simulink model "MiMo_Sim"  (R2014a)
settings: Solver=ode45  StartTime=0.0  StopTime=10.0  RelTol=1e-3
values from neighbouring files (symbols this model uses):
  A = ee661_proj3_ss_model.A    [Untitled.m]
  B = ee661_proj3_ss_model.B    [Untitled.m]
  C = ee661_proj3_ss_model.C    [Untitled.m]
  D = ee661_proj3_ss_model.D    [Untitled.m]
  r = length(v{x}) - length(u{x})    [MIMOTest.m]
undefined symbols (not defined in the file or in its folder): initialConditions
settings Model: Creator=Aaron  LastModifiedBy=Aaron

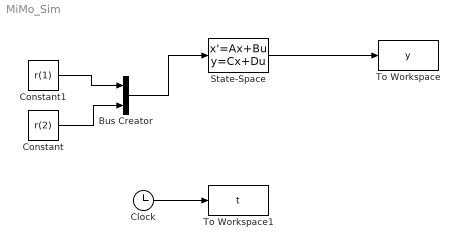
== system MiMo_Sim ==
  Bus Creator : BusCreator  Inputs=2
  Clock : Clock
  Constant : Constant  Value=r(2)
  Constant1 : Constant  Value=r(1)
  State-Space : StateSpace  A=A  B=B  C=C  D=D  X0=initialConditions
  To Workspace : ToWorkspace  VariableName=y  SampleTime=-1
  To Workspace1 : ToWorkspace  VariableName=t  SampleTime=-1
  wires:
  State-Space/1 -> To Workspace/1
  Clock/1 -> To Workspace1/1
  Constant1/1 -> Bus Creator/1
  Constant/1 -> Bus Creator/2
  Bus Creator/1 -> State-Space/1
